simulink model "OPC_Server_simulink_example"  (R2020a)
settings: Solver=VariableStepAuto  StartTime=0.0  StopTime=25  RelTol=1e-3
libraries: opclib x3
settings Model: Creator=Jonas  LastModifiedBy=Jonas

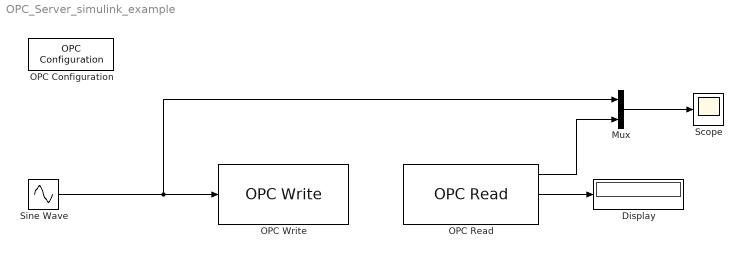
== system OPC_Server_simulink_example ==
  Display : Display
  Mux : Mux  Inputs=3
  OPC Configuration : opclib/OPC Configuration  opcServers=localhost/Matrikon.OPC.Simulation.1/10  errMissingItems=Error  errReadWrite=Warn  errShutdown=Error  errRTViolation=Warn  rtEnable=on  speedup=1  showLatency=off  beingUsed=on
      settings: SourceProductBaseCode=OT
  OPC Read : opclib/OPC Read  serverHost=localhost  serverID=Matrikon.OPC.Simulation.1  itemIDs=Bucket Brigade.Real8  readMode=Synchronous (cache)  dataType=double  updateRate=0.5  showQual=on  showTS=on  tsMode=Seconds since start
      settings: SourceProductBaseCode=OT
  OPC Write : opclib/OPC Write  serverHost=localhost  serverID=Matrikon.OPC.Simulation.1  itemIDs=Bucket Brigade.Real8  writeMode=Synchronous  updateRate=0
      settings: SourceProductBaseCode=OT
  Scope : Scope
  Sine Wave : Sin  Frequency=.25  SampleTime=0
  wires:
  Sine Wave/1 -> Mux/1, OPC Write/1
  OPC Read/1 -> Mux/3
  Mux/1 -> Scope/1
  OPC Read/2 -> Display/1
